simulink model "EkalmanF_ac_sim"  (R2025b)
settings: Solver=VariableStepAuto  StartTime=0.0  StopTime=StopTime  RelTol=1e-3
values from neighbouring files (symbols this model uses):
  B = single([0.5*dt^2 0; 0 0.5*dt^2; dt 0; 0 dt])    [kalman_ac.m]
  C = eye(4)/(H*H' + R)    [kalman_ac.m]
  dt = 0.02    [kalman_ac.m]
  H = single(diag([1,1,1,1]))    [kalman_ac.m]
  Q = single(0.1 * eye(4))    [kalman_ac.m]
  time = single(0:dt:StopTime)    [kalman_ac.m]
undefined symbols (not defined in the file or in its folder): T1, T10, T11, T12, T13, T14, T15, T16, T2, T3, T4, T5, T6, T7, T8, T9
libraries: hdlsllib x3, dspsrcs4 x3
settings Model: Creator=stefa  LastModifiedBy=david
settings OptimizationCC: BlockReduction=off  ConditionallyExecuteInputs=off

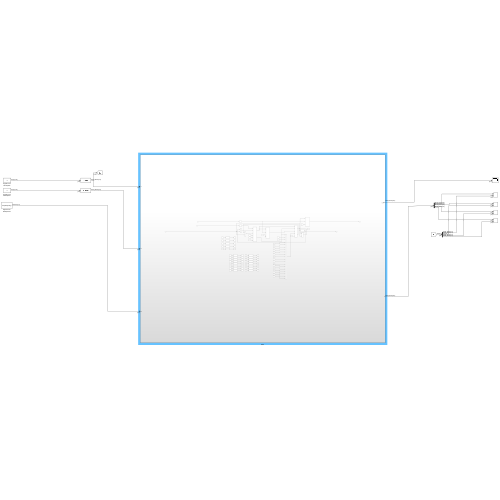
[thumbnail: Simulink's stored preview of the top-level diagram]
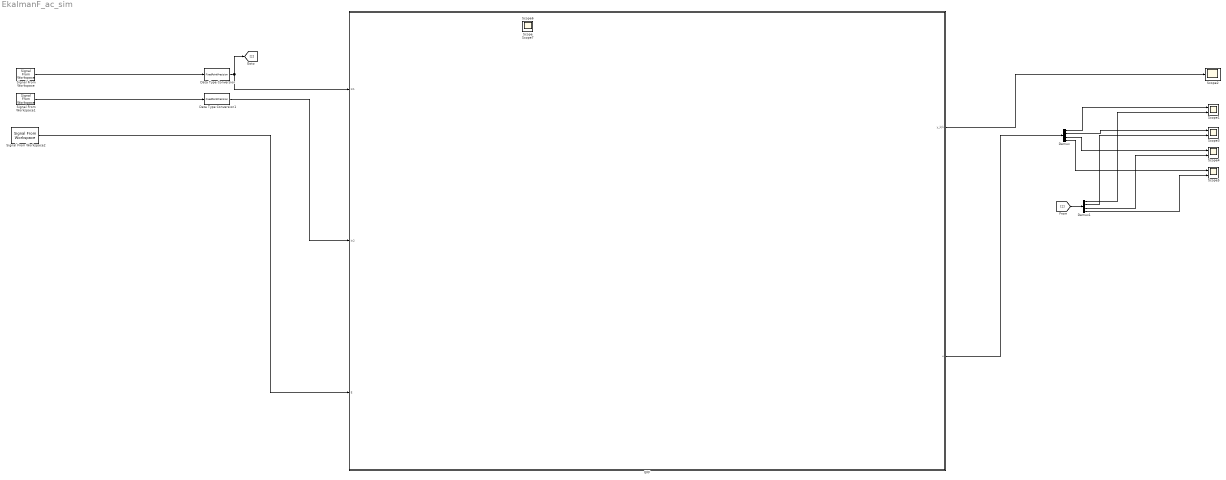
== system EkalmanF_ac_sim ==
  Data Type Conversion : DataTypeConversion  OutMin=[1e-3]  OutMax=[1000]  OutDataTypeStr=FixedPointPrecision  SaturateOnIntegerOverflow=off  RndMeth=Floor
  Data Type Conversion1 : DataTypeConversion  OutDataTypeStr=FixedPointPrecision  SaturateOnIntegerOverflow=off  RndMeth=Floor
  Demux : Demux
  Demux1 : Demux
  EKF : Subsystem
  Scope{1,3..5} (4 alike) : Scope  NumInputPorts=2
      Scope1 settings: ActiveDisplayYMinimum=-0.86714764326171867  ActiveDisplayYMaximum=2.8586929351527814  DataLoggingSaveFormat=Array
      Scope3 settings: ActiveDisplayYMinimum=-3.2632629487193681  ActiveDisplayYMaximum=3.9620158516637924  DataLoggingVariableName=ScopeData2  DataLoggingSaveFormat=Array
      Scope4 settings: ActiveDisplayYMinimum=-5.84392599463885  ActiveDisplayYMaximum=2.7669674927194179  DataLoggingVariableName=ScopeData3  DataLoggingSaveFormat=Array
      Scope5 settings: ActiveDisplayYMinimum=-5.0260366041316269  ActiveDisplayYMaximum=3.5090934704886196  DataLoggingVariableName=ScopeData4  DataLoggingSaveFormat=Array
  Scope{,2,6..7} (4 alike) : Scope
      Scope2 settings: ActiveDisplayYMinimum=-1.1122805343511448  ActiveDisplayYMaximum=1.0927194656488552  DataLoggingSaveFormat=Array
      Scope settings: ActiveDisplayYMinimum=-9.1353842219735029  ActiveDisplayYMaximum=57.624373102579447  DataLoggingVariableName=ScopeData5
      Scope6 settings: ActiveDisplayYMinimum=-1  ActiveDisplayYMaximum=1  DataLoggingVariableName=ScopeData6
      Scope7 settings: ActiveDisplayYMinimum=-0.035523056983947747  ActiveDisplayYMaximum=0.31970751285552979  DataLoggingVariableName=ScopeData7
  Signal From Workspace : dspsrcs4/Signal From Workspace  X=z  Ts=dt  nsamps=1  OutputAfterFinalValue=Setting to zero  ignoreOrWarnInputAndFrameLengths=off  OutputFrames=off
  Signal From Workspace1 : dspsrcs4/Signal From Workspace  X=u  Ts=dt  nsamps=1  OutputAfterFinalValue=Setting to zero  ignoreOrWarnInputAndFrameLengths=off  OutputFrames=off
  Signal From Workspace2 : dspsrcs4/Signal From Workspace  X=true(size(time))  Ts=dt  nsamps=1  OutputAfterFinalValue=Setting to zero  ignoreOrWarnInputAndFrameLengths=off  OutputFrames=off
  wires:
  Signal From Workspace1/1 -> Data Type Conversion1/1
  Signal From Workspace/1 -> Data Type Conversion/1
  Demux/1 -> Scope1/1
  Demux/2 -> Scope3/1
  Demux/3 -> Scope4/1
  Demux/4 -> Scope5/1
  [z] -> Demux1/1
  Demux1/1 -> Scope1/2
  Demux1/2 -> Scope3/2
  Demux1/3 -> Scope4/2
  Demux1/4 -> Scope5/2
  Data Type Conversion/1 -> EKF/1(In1), [z]
  Data Type Conversion1/1 -> EKF/2(In2)
  Signal From Workspace2/1 -> EKF/3(E)
  EKF/1(y_k|k) -> Scope2/1
  EKF/2(u) -> Demux/1

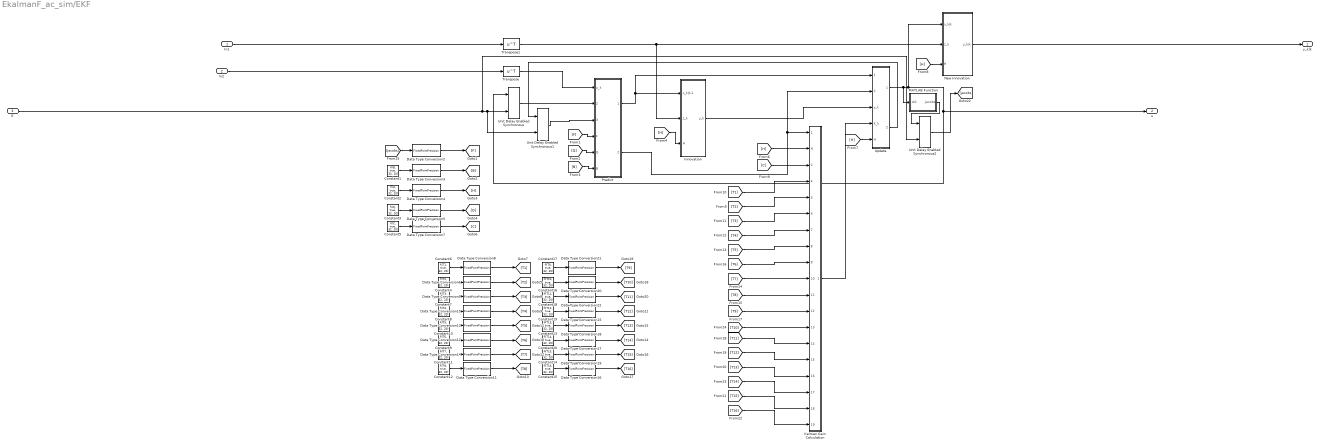
== system EkalmanF_ac_sim/EKF ==
  In1 : Inport
  In2 : Inport  Port=2
  E : Inport  Port=3
  Constant1 : Constant  Value=fi(B, true, 32, 20)
  Constant10 : Constant  Value=fi(T5, true, 32, 20)
  Constant11 : Constant  Value=fi(T7, true, 32, 20)
  Constant12 : Constant  Value=fi(T8, true, 32, 20)
  Constant13 : Constant  Value=fi(T13, true, 32, 20)
  Constant14 : Constant  Value=fi(T15, true, 32, 20)
  Constant15 : Constant  Value=fi(T16, true, 32, 20)
  Constant16 : Constant  Value=fi(T10, true, 32, 20)
  Constant17 : Constant  Value=fi(T9, true, 32, 20)
  Constant18 : Constant  Value=fi(T11, true, 32, 20)
  Constant19 : Constant  Value=fi(T12, true, 32, 20)
  Constant2 : Constant  Value=fi(H, true, 32, 20)
  Constant20 : Constant  Value=fi(T14, true, 32, 20)
  Constant3 : Constant  Value=fi(Q, true, 32, 20)
  Constant4 : Constant  Value=fi(T2, true, 32, 20)
  Constant5 : Constant  Value=fi(C, true, 32, 20)
  Constant6 : Constant  Value=fi(T1, true, 32, 20)
  Constant7 : Constant  Value=fi(T3, true, 32, 20)
  Constant8 : Constant  Value=fi(T4, true, 32, 20)
  Constant9 : Constant  Value=fi(T6, true, 32, 20)
  Data Type Conversion{2..22} (21 alike) : DataTypeConversion  OutDataTypeStr=FixedPointPrecision  SaturateOnIntegerOverflow=off  RndMeth=Floor
  Innovation : Subsystem
  Kalman Gain Calculation : Subsystem
  MATLAB Function : MATLAB Function  TreatAsAtomicUnit=on
  New Innovation : Subsystem
  Predict : Subsystem
  Transpose : Math  Operator=transpose  SignedPower=on  RndMeth=Zero
  Transpose1 : Math  Operator=transpose  SignedPower=on  RndMeth=Zero
  Unit Delay Enabled Synchronous : hdlsllib/Discrete/Unit Delay Enabled Synchronous  InitialCondition=0.0  SampleTime=-1
  Unit Delay Enabled Synchronous1 : hdlsllib/Discrete/Unit Delay Enabled Synchronous  InitialCondition=0.0  SampleTime=-1
  Unit Delay Enabled Synchronous2 : hdlsllib/Discrete/Unit Delay Enabled Synchronous  InitialCondition=0.0  SampleTime=-1
  Update : Subsystem
  y_k|k : Outport
  u : Outport  Port=2
  wires:
  Constant19/1 -> Data Type Conversion15/1
  Constant12/1 -> Data Type Conversion11/1
  Data Type Conversion15/1 -> [T12]
  Data Type Conversion6/1 -> [T2]
  E/1 -> Unit Delay Enabled Synchronous2/2, Unit Delay Enabled Synchronous/2, Unit Delay Enabled Synchronous1/2
  Transpose/1 -> Predict/1(u_k)
  Predict/1(x_k|k-1) -> Update/1(x_k|k-1), Innovation/1(x_k|k-1)
  Data Type Conversion20/1 -> [T10]
  Constant4/1 -> Data Type Conversion6/1
  Unit Delay Enabled Synchronous/1 -> Predict/2(x_k-1|k-1)
  Constant18/1 -> Data Type Conversion22/1
  Data Type Conversion8/1 -> [T1]
  In2/1 -> Transpose/1
  [T4] -> Kalman Gain Calculation/7(T4)
  Update/1(x_k|k) -> MATLAB Function/1(xkk), New Innovation/1(x_k|k), u/1, Unit Delay Enabled Synchronous/1
  Constant14/1 -> Data Type Conversion19/1
  MATLAB Function/1(Jacobs) -> Unit Delay Enabled Synchronous2/1
  Constant9/1 -> Data Type Conversion12/1
  Data Type Conversion5/1 -> [Q]
  [T14] -> Kalman Gain Calculation/17(T14)
  Data Type Conversion4/1 -> [H]
  Data Type Conversion16/1 -> [T16]
  [T2] -> Kalman Gain Calculation/5(T2)
  Constant16/1 -> Data Type Conversion20/1
  Constant6/1 -> Data Type Conversion8/1
  Constant17/1 -> Data Type Conversion21/1
  [T7] -> Kalman Gain Calculation/10(T7)
  [H] -> Innovation/3(H)
  Data Type Conversion12/1 -> [T6]
  [Q] -> Predict/5(Q)
  Constant1/1 -> Data Type Conversion3/1
  [T3] -> Kalman Gain Calculation/6(T3)
  [T6] -> Kalman Gain Calculation/9(T6)
  Constant3/1 -> Data Type Conversion5/1
  Innovation/1(y_k) -> Update/3(y_k)
  Data Type Conversion2/1 -> [F]
  [B] -> Predict/6(B)
  Data Type Conversion21/1 -> [T9]
  Constant20/1 -> Data Type Conversion17/1
  [Jacobs] -> Data Type Conversion2/1
  Data Type Conversion13/1 -> [T5]
  Constant15/1 -> Data Type Conversion16/1
  [H] -> New Innovation/3(H)
  [T15] -> Kalman Gain Calculation/18(T15)
  Unit Delay Enabled Synchronous1/1 -> Predict/3(P_k-1|k-1)
  Data Type Conversion11/1 -> [T8]
  Constant10/1 -> Data Type Conversion13/1
  [T9] -> Kalman Gain Calculation/12(T9)
  Kalman Gain Calculation/1(K_k) -> Update/4(K_k)
  Data Type Conversion10/1 -> [T4]
  [T8] -> Kalman Gain Calculation/11(T8)
  [T5] -> Kalman Gain Calculation/8(T5)
  Data Type Conversion14/1 -> [T7]
  Data Type Conversion3/1 -> [B]
  Data Type Conversion17/1 -> [T14]
  [F] -> Predict/4(F)
  Data Type Conversion18/1 -> [T13]
  Data Type Conversion7/1 -> [C]
  Data Type Conversion19/1 -> [T15]
  Constant7/1 -> Data Type Conversion9/1
  [H] -> Update/5(H)
  Constant5/1 -> Data Type Conversion7/1
  [T11] -> Kalman Gain Calculation/14(T11)
  [T1] -> Kalman Gain Calculation/4(T1)
  [C] -> Kalman Gain Calculation/3(C)
  Constant11/1 -> Data Type Conversion14/1
  Predict/2(P_k|k-1) -> Update/2(P_k|k-1), Kalman Gain Calculation/1(P_k|k-1)
  Update/2(P_k|k) -> Unit Delay Enabled Synchronous1/1
  Constant13/1 -> Data Type Conversion18/1
  [T16] -> Kalman Gain Calculation/19(T16)
  Data Type Conversion22/1 -> [T11]
  Transpose1/1 -> Innovation/2(z_k), New Innovation/2(z_k)
  Unit Delay Enabled Synchronous2/1 -> [Jacobs]
  [T10] -> Kalman Gain Calculation/13(T10)
  Constant8/1 -> Data Type Conversion10/1
  [H] -> Kalman Gain Calculation/2(H)
  Constant2/1 -> Data Type Conversion4/1
  [T12] -> Kalman Gain Calculation/15(T12)
  Data Type Conversion9/1 -> [T3]
  [T13] -> Kalman Gain Calculation/16(T13)
  New Innovation/1(y_k|k) -> y_k|k/1
  In1/1 -> Transpose1/1

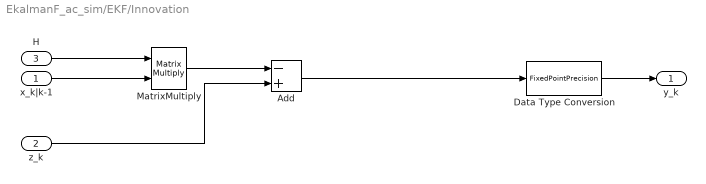
== system EkalmanF_ac_sim/EKF/Innovation ==
  x_k|k-1 : Inport
  z_k : Inport  Port=2
  H : Inport  Port=3
  Add : Sum  Inputs=-+
  Data Type Conversion : DataTypeConversion  OutDataTypeStr=FixedPointPrecision  SaturateOnIntegerOverflow=off  RndMeth=Floor
  MatrixMultiply : Product  Multiplication=Matrix(*)
  y_k : Outport
  wires:
  x_k|k-1/1 -> MatrixMultiply/2
  MatrixMultiply/1 -> Add/1
  z_k/1 -> Add/2
  Add/1 -> Data Type Conversion/1
  H/1 -> MatrixMultiply/1
  Data Type Conversion/1 -> y_k/1

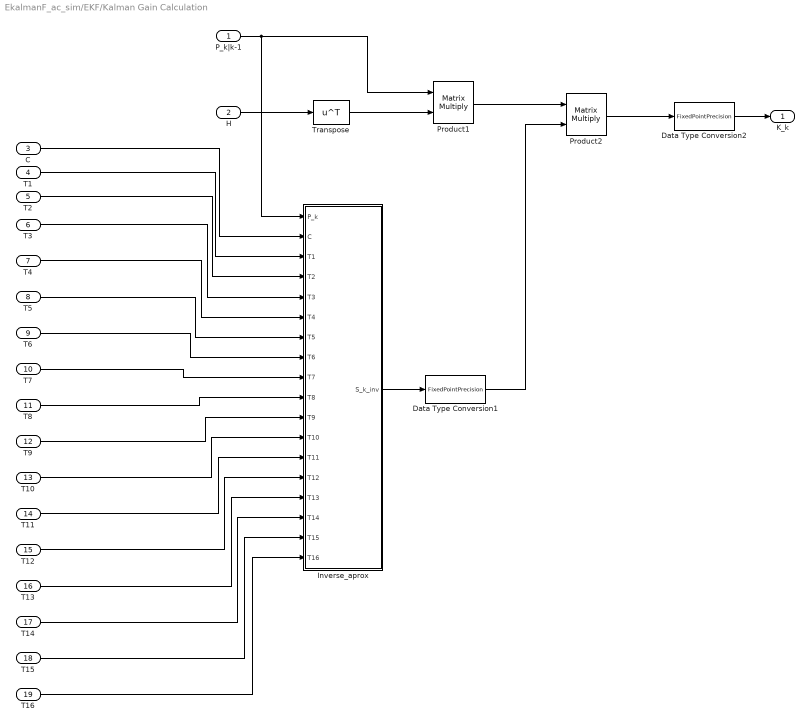
== system EkalmanF_ac_sim/EKF/Kalman Gain Calculation ==
  P_k|k-1 : Inport
  H : Inport  Port=2
  C : Inport  Port=3
  T1 : Inport  Port=4
  T2 : Inport  Port=5
  T3 : Inport  Port=6
  T4 : Inport  Port=7
  T5 : Inport  Port=8
  T6 : Inport  Port=9
  T7 : Inport  Port=10
  T8 : Inport  Port=11
  T9 : Inport  Port=12
  T10 : Inport  Port=13
  T11 : Inport  Port=14
  T12 : Inport  Port=15
  T13 : Inport  Port=16
  T14 : Inport  Port=17
  T15 : Inport  Port=18
  T16 : Inport  Port=19
  Data Type Conversion1 : DataTypeConversion  OutDataTypeStr=FixedPointPrecision  SaturateOnIntegerOverflow=off  RndMeth=Floor
  Data Type Conversion2 : DataTypeConversion  OutDataTypeStr=FixedPointPrecision  SaturateOnIntegerOverflow=off  RndMeth=Floor
  Inverse_aprox : MATLAB Function  TreatAsAtomicUnit=on
  Product1 : Product  Multiplication=Matrix(*)
  Product2 : Product  Multiplication=Matrix(*)
  Transpose : Math  Operator=transpose  SignedPower=on  RndMeth=Zero
  K_k : Outport
  wires:
  H/1 -> Transpose/1
  P_k|k-1/1 -> Product1/1, Inverse_aprox/1(P_k)
  Transpose/1 -> Product1/2
  Inverse_aprox/1(S_k_inv) -> Data Type Conversion1/1
  Product2/1 -> Data Type Conversion2/1
  Product1/1 -> Product2/1
  Data Type Conversion1/1 -> Product2/2
  Data Type Conversion2/1 -> K_k/1
  C/1 -> Inverse_aprox/2(C)
  T1/1 -> Inverse_aprox/3(T1)
  T2/1 -> Inverse_aprox/4(T2)
  T3/1 -> Inverse_aprox/5(T3)
  T4/1 -> Inverse_aprox/6(T4)
  T5/1 -> Inverse_aprox/7(T5)
  T6/1 -> Inverse_aprox/8(T6)
  T7/1 -> Inverse_aprox/9(T7)
  T8/1 -> Inverse_aprox/10(T8)
  T9/1 -> Inverse_aprox/11(T9)
  T10/1 -> Inverse_aprox/12(T10)
  T11/1 -> Inverse_aprox/13(T11)
  T12/1 -> Inverse_aprox/14(T12)
  T13/1 -> Inverse_aprox/15(T13)
  T14/1 -> Inverse_aprox/16(T14)
  T15/1 -> Inverse_aprox/17(T15)
  T16/1 -> Inverse_aprox/18(T16)

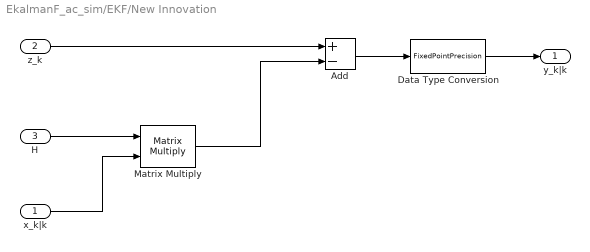
== system EkalmanF_ac_sim/EKF/New Innovation ==
  x_k|k : Inport
  z_k : Inport  Port=2
  H : Inport  Port=3
  Add : Sum  Inputs=+-
  Data Type Conversion : DataTypeConversion  OutDataTypeStr=FixedPointPrecision  SaturateOnIntegerOverflow=off  RndMeth=Floor
  Matrix Multiply : Product  Multiplication=Matrix(*)
  y_k|k : Outport
  wires:
  z_k/1 -> Add/1
  H/1 -> Matrix Multiply/1
  x_k|k/1 -> Matrix Multiply/2
  Matrix Multiply/1 -> Add/2
  Add/1 -> Data Type Conversion/1
  Data Type Conversion/1 -> y_k|k/1

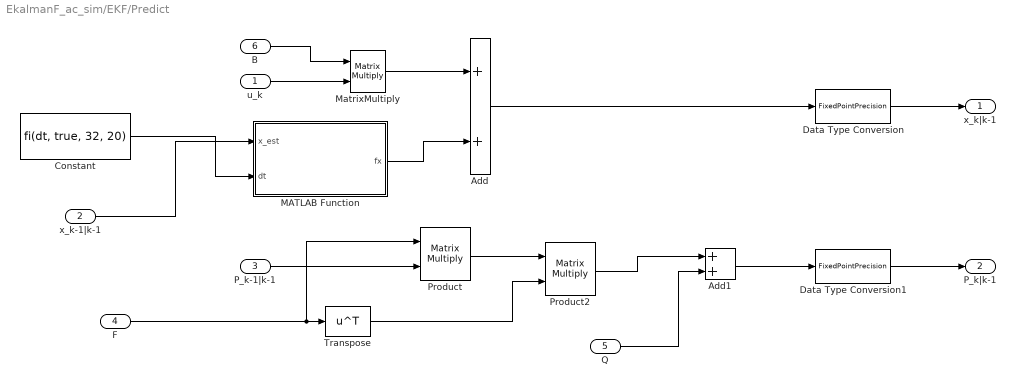
== system EkalmanF_ac_sim/EKF/Predict ==
  u_k : Inport
  x_k-1|k-1 : Inport  Port=2
  P_k-1|k-1 : Inport  Port=3
  F : Inport  Port=4
  Q : Inport  Port=5
  B : Inport  Port=6
  Add : Sum
  Add1 : Sum
  Constant : Constant  Value=fi(dt, true, 32, 20)
  Data Type Conversion : DataTypeConversion  OutDataTypeStr=FixedPointPrecision  SaturateOnIntegerOverflow=off  RndMeth=Floor
  Data Type Conversion1 : DataTypeConversion  OutDataTypeStr=FixedPointPrecision  SaturateOnIntegerOverflow=off  RndMeth=Floor
  MATLAB Function : MATLAB Function  TreatAsAtomicUnit=on
  MatrixMultiply : Product  Multiplication=Matrix(*)
  Product : Product  Multiplication=Matrix(*)
  Product2 : Product  Multiplication=Matrix(*)
  Transpose : Math  Operator=transpose  SignedPower=on  RndMeth=Zero
  x_k|k-1 : Outport
  P_k|k-1 : Outport  Port=2
  wires:
  x_k-1|k-1/1 -> MATLAB Function/1(x_est)
  Add/1 -> Data Type Conversion/1
  MatrixMultiply/1 -> Add/1
  P_k-1|k-1/1 -> Product/2
  Q/1 -> Add1/2
  Add1/1 -> Data Type Conversion1/1
  Product2/1 -> Add1/1
  Product/1 -> Product2/1
  Transpose/1 -> Product2/2
  B/1 -> MatrixMultiply/1
  F/1 -> Transpose/1, Product/1
  Data Type Conversion/1 -> x_k|k-1/1
  Data Type Conversion1/1 -> P_k|k-1/1
  u_k/1 -> MatrixMultiply/2
  MATLAB Function/1(fx) -> Add/2
  Constant/1 -> MATLAB Function/2(dt)

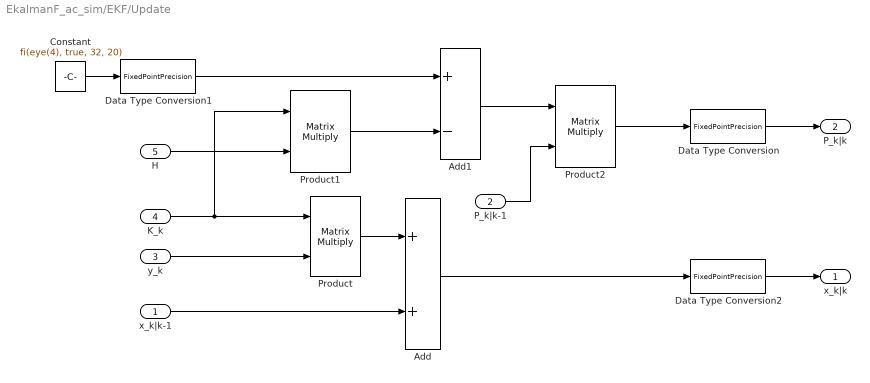
== system EkalmanF_ac_sim/EKF/Update ==
  x_k|k-1 : Inport
  P_k|k-1 : Inport  Port=2
  y_k : Inport  Port=3
  K_k : Inport  Port=4
  H : Inport  Port=5
  Add : Sum
  Add1 : Sum  Inputs=+-
  Constant : Constant  Value=fi(eye(4), true, 32, 20)
  Data Type Conversion : DataTypeConversion  OutDataTypeStr=FixedPointPrecision  SaturateOnIntegerOverflow=off  RndMeth=Floor
  Data Type Conversion1 : DataTypeConversion  OutDataTypeStr=FixedPointPrecision  SaturateOnIntegerOverflow=off  RndMeth=Floor
  Data Type Conversion2 : DataTypeConversion  OutDataTypeStr=FixedPointPrecision  SaturateOnIntegerOverflow=off  RndMeth=Floor
  Product : Product  Multiplication=Matrix(*)
  Product1 : Product  Multiplication=Matrix(*)
  Product2 : Product  Multiplication=Matrix(*)
  x_k|k : Outport
  P_k|k : Outport  Port=2
  wires:
  K_k/1 -> Product1/1, Product/1
  y_k/1 -> Product/2
  Product/1 -> Add/1
  x_k|k-1/1 -> Add/2
  Add/1 -> Data Type Conversion2/1
  H/1 -> Product1/2
  Product1/1 -> Add1/2
  Constant/1 -> Data Type Conversion1/1
  P_k|k-1/1 -> Product2/2
  Add1/1 -> Product2/1
  Product2/1 -> Data Type Conversion/1
  Data Type Conversion1/1 -> Add1/1
  Data Type Conversion/1 -> P_k|k/1
  Data Type Conversion2/1 -> x_k|k/1

== matlab function EkalmanF_ac_sim/EKF/MATLAB Function ==
  data: xkk input; Jacobs output
function Jacobs = fcn(xkk)
%#codegen
    % 1. Math Rules (Keep 'Zero' rounding)
    F = fimath('RoundingMethod', 'Zero', ...
               'OverflowAction', 'Wrap', ...
               'ProductMode', 'FullPrecision', ...
               'SumMode', 'FullPrecision');
    xkk = setfimath(xkk, F);

    % 2. Pre-allocate output
    Jacobs = zeros(4, 4, 'like', xkk);

    % 3. Constants
    c_one  = cast(1.0,  'like', xkk);
    c_0p3  = cast(0.3,  'like', xkk);
    c_0p02 = cast(0.02, 'like', xkk);

    % 4. Calculate terms using our CUSTOM approximation function
    % This bypasses the built-in 'cos' and its division logic entirely.
    term1 = c_one + c_0p3 * cos_approx(xkk(1));
    term2 = c_one + c_0p3 * cos_approx(xkk(2));

    % 5. Assign
    Jacobs(1,1) = term1;
    Jacobs(1,3) = c_0p02;
    Jacobs(2,2) = term2;
    Jacobs(2,4) = c_0p02;
    Jacobs(3,3) = c_one;
    Jacobs(4,4) = c_one;
end

% --- SUB-FUNCTION: Hardware Friendly Cosine ---
function y = cos_approx(theta)
    % 4th-Order Taylor Series: 1 - x^2/2 + x^4/24
    % Valid for range: -pi/2 to +pi/2
    % Uses only MULT and ADD (No Division!)
    
    % Define coefficients with same type as input
    c1 = cast(1.0,         'like', theta);
    c2 = cast(0.5,         'like', theta); % 1/2
    c3 = cast(0.04166666,  'like', theta); % 1/24

    % Calculations
    theta2 = theta * theta;      % x^2
    theta4 = theta2 * theta2;    % x^4
    
    % Result: 1 - 0.5*x^2 + 0.0416*x^4
    y = c1 - (c2 * theta2) + (c3 * theta4);
end

== matlab function EkalmanF_ac_sim/EKF/Kalman Gain Calculation/Inverse_aprox ==
  data: S_k_inv output; P_k input; C input; T1 input; T2 input; T3 input; T4 input; T5 input; T6 input; T7 input; T8 input; T9 input; T10 input; T11 input; T12 input; T13 input; T14 input; T15 input; T16 input
function S_k_inv = inverse_aprox(P_k, C, T1, T2, T3, T4, T5, T6, T7, T8, T9, T10, T11, T12, T13, T14, T15, T16)
    Z = P_k - fi(eye(4),true, 66, 40);
    sum = fi(zeros(4,4),true, 66, 40);
    sum = sum + T1*Z(1,1);
    sum = sum + T2*Z(1,2);
    sum = sum + T3*Z(1,3);
    sum = sum + T4*Z(1,4);
    sum = sum + T5*Z(2,1);
    sum = sum + T6*Z(2,2);
    sum = sum + T7*Z(2,3);
    sum = sum + T8*Z(2,4);
    sum = sum + T9*Z(3,1);
    sum = sum + T10*Z(3,2);
    sum = sum + T11*Z(3,3);
    sum = sum + T12*Z(3,4);
    sum = sum + T13*Z(4,1);
    sum = sum + T14*Z(4,2);
    sum = sum + T15*Z(4,3);
    sum = sum + T16*Z(4,4);    
    S_k_inv = C - fi(sum, true, 32, 20);
end

== matlab function EkalmanF_ac_sim/EKF/Predict/MATLAB Function ==
  data: x_est input; fx output; dt input
function fx = state_transition_fcn(x_est, dt)
%#codegen
    
    % 1. Define Fixed-Point Math Properties
    % CRITICAL: 'Saturate' is safer for control systems than 'Wrap'.
    % We use 'KeepLSB' or specific lengths to prevent bit-width explosion.
    F = fimath('RoundingMethod', 'Floor', ...
               'OverflowAction', 'Saturate', ...
               'ProductMode', 'SpecifyPrecision', ...
               'ProductWordLength', 32, ...
               'ProductFractionLength', 24, ...
               'SumMode', 'SpecifyPrecision', ...
               'SumWordLength', 32, ...
               'SumFractionLength', 24);
           
    % Apply fimath to inputs to ensure internal ops use these rules
    x_est = setfimath(x_est, F);
    dt    = setfimath(dt, F);

    % 2. Pre-allocate output
    fx = zeros(4, 1, 'like', x_est);
    
    % 3. Constants
    c_0p3 = cast(0.3, 'like', x_est);

    % 4. Compute State Equations
    % We process indices 1 and 2 in a loop. HDL Coder can interpret this 
    % to either share resources (save space) or unroll (save time).
    for i = 1:2
        % Calculate Sine Term using optimized function
        sin_val = sin_approx_horner(x_est(i));
        
        % x[k] + x[k+2]*dt + 0.3*sin(x[k])
        % Note: explicitly casting the multiply result helps HDL Coder
        term_dt  = x_est(i+2) * dt;
        term_sin = c_0p3 * sin_val;
        
        fx(i) = x_est(i) + term_dt + term_sin;
    end

    % Pass through remaining states
    fx(3) = x_est(3);
    fx(4) = x_est(4);
end

% --- SUB-FUNCTION: Optimized Sine (Horner's Method) ---
function y = sin_approx_horner(theta)
    % Uses Horner's Rule to reduce the number of multipliers.
    % Original: x - c2*x^3 + c3*x^5
    % Horner's: x * (1 - x^2 * (c2 - c3*x^2))
    
    % Define coefficients
    % c2 = 1/6  = 0.16666666...
    % c3 = 1/120 = 0.00833333...
    c2 = cast(0.16666667, 'like', theta); 
    c3 = cast(0.00833333, 'like', theta);
    c1 = cast(1.0,        'like', theta);

    % 1. Calculate x^2 once
    theta_sq = theta * theta;

    % 2. Inner term: (c2 - c3 * theta^2)
    inner_term = c2 - (c3 * theta_sq);

    % 3. Middle term: 1 - theta^2 * (inner)
    mid_term = c1 - (theta_sq * inner_term);

    % 4. Final result: theta * mid_term
    y = theta * mid_term;
end
